simulink model "lab2"  (R2014a)
settings: Solver=ode45  StartTime=0.0  StopTime=0.1  RelTol=1e-3
libraries: powerlib x11, powerlib_meascontrol x10
settings Model: Creator=Thodoris  LastModifiedBy=Thodoris

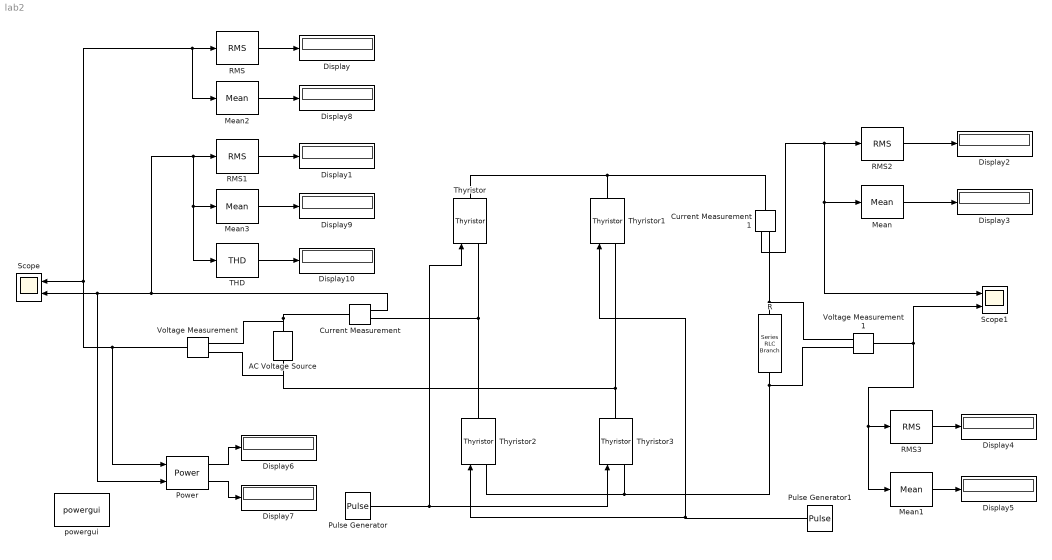
== system lab2 ==
  AC Voltage Source : powerlib/Electrical Sources/AC Voltage Source  Amplitude=50*sqrt(2)  Phase=0  Frequency=50  SampleTime=0  Measurements=None
  Current Measurement : powerlib/Measurements/Current Measurement  PhasorSimulation=off  OutputType=Complex  PSBequivalent=0
  Current Measurement1 : powerlib/Measurements/Current Measurement  PhasorSimulation=off  OutputType=Complex  PSBequivalent=0
  Display{,1..10} (11 alike) : Display
  Mean{,1..3} (4 alike) : powerlib_meascontrol/Measurements/Mean  Freq=50  Vinit=0  Ts=0
  Power : powerlib_meascontrol/Measurements/Power  Freq=60  Vinit=[1, 0]  Iinit=[1, 0]  Ts=0
  Pulse Generator : DiscretePulseGenerator  PulseType=Time based  Period=0.02  PulseWidth=5  PhaseDelay=0.02/4
  Pulse Generator1 : DiscretePulseGenerator  PulseType=Time based  Period=0.02  PulseWidth=5  PhaseDelay=0.01 + 0.02/4
  R : powerlib/Elements/Series RLC Branch  LConnTagsString=__new0  RConnTagsString=__new0  BranchType=R  Resistance=50.8  Inductance=150e-3  SetiL0=off  InitialCurrent=0  Capacitance=1e-6  Setx0=off  InitialVoltage=0  Measurements=None
  RMS{,1..3} (4 alike) : powerlib_meascontrol/Measurements/RMS  TrueRMS=on  Freq=50  RMSInit=120  Ts=0
  Scope : Scope  NumInputPorts=2
      settings: YMin=-5~-5  YMax=5~5
  Scope1 : Scope  NumInputPorts=2
      settings: YMin=-5~-5  YMax=5~5
  THD : powerlib_meascontrol/Measurements/THD  Freq=60  Ts=0
  Thyristor{,1..3} (4 alike) : powerlib/Power Electronics/Thyristor  Ron=0.001  Lon=0  Vf=0.8  IC=0  Rs=500  Cs=250e-9  Measurements=off
  Voltage Measurement : powerlib/Measurements/Voltage Measurement  PhasorSimulation=off  OutputType=Complex  PSBequivalent=0
  Voltage Measurement1 : powerlib/Measurements/Voltage Measurement  PhasorSimulation=off  OutputType=Complex  PSBequivalent=0
  powergui : powerlib/powergui  Priority=1  SimulationMode=Continuous  SolverType=Tustin  SampleTime=50e-6  frequency=60  SPID=off  DisableSnubberDevices=off  DisableRonSwitches=off  DisableVfSwitches=off  SwTol=0  Interpol=off  DisplayEquations=off  Ts=0  methode=off  frequencyindice=50  Pbase=100e6  ErrMax=1e-4  Iterations=50  UnitsV=kV  UnitsW=MW  FunctionMessages=off  echomessages=off  HookPort=off  EnableUseOfTLC=off  x0status=blocks  RestoreLinks=warning  ResistiveCurrentMeasurement=off  Frange=[0:2:500]  Ylog=off  Xlog=on  ShowGrid=off  save=off  variable=ZData  structure=0  ZoomFFT=off  StartTime=0.0  cycles=1  DisplayStyle=1  fundamental=60  FreqAxis=off  MaxFrequency=1000  frequencyindicesteady=1  RmsSteady=1  display=off
  wires:
  RMS/1 -> Display/1
  RMS1/1 -> Display1/1
  Voltage Measurement/1 -> Power/1, Scope/1, Mean2/1, RMS/1
  Voltage Measurement1/1 -> Scope1/2, RMS3/1, Mean1/1
  Current Measurement1/1 -> Mean/1, Scope1/1, RMS2/1
  RMS2/1 -> Display2/1
  Mean/1 -> Display3/1
  RMS3/1 -> Display4/1
  Mean1/1 -> Display5/1
  Power/1 -> Display6/1
  Power/2 -> Display7/1
  Pulse Generator/1 -> Thyristor3/1, Thyristor/1
  Pulse Generator1/1 -> Thyristor2/1, Thyristor1/1
  Mean2/1 -> Display8/1
  Current Measurement/1 -> THD/1, Mean3/1, RMS1/1, Power/2, Scope/2
  Mean3/1 -> Display9/1
  THD/1 -> Display10/1
  connections:
  Thyristor1/RConn1 -- Current Measurement1/LConn1 -- Thyristor/RConn1
  Thyristor2/LConn1 -- Thyristor3/LConn1 -- Voltage Measurement1/LConn2 -- R/RConn1
  Thyristor3/RConn1 -- AC Voltage Source/LConn1 -- Voltage Measurement/LConn2 -- Thyristor1/LConn1
  AC Voltage Source/RConn1 -- Current Measurement/LConn1 -- Voltage Measurement/LConn1
  Thyristor2/RConn1 -- Thyristor/LConn1 -- Current Measurement/RConn1
  Voltage Measurement1/LConn1 -- Current Measurement1/RConn1 -- R/LConn1
